simulink model "es2sim"  (R2023b)
settings: Solver=VariableStepAuto  StartTime=0.0  StopTime=200  RelTol=1e-3
values from neighbouring files (symbols this model uses):
  d = 0    [es2.m]
  ea0 = [0 0.3927 0]'    [es2.m]
  ea_dot_ref = [0.001745 0 0.04859]'    [es2.m]
  IJ = inv(J)    [es1.m]    (also in es2.m)
  J = diag([10000,9000,12000])    [es1.m]    (also in es2.m = [399 -2.81 -1.31)
  q0 = [0.6853,0.6953,0.1531,0.1531]'    [es1.m]    (also in es2.m = [0 0 1 0]')
  w0 = [0.53, 0.53,0.053]'    [es1.m]    (also in es2.m = [0.1 -0.9 0.12]')
libraries: vrlib x1
settings Model: Creator=luigi  LastModifiedBy=luigi

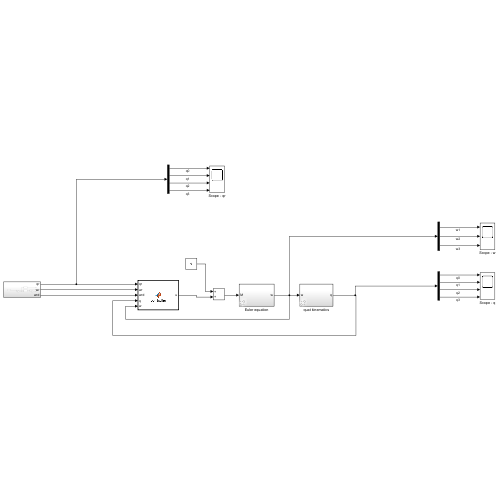
[thumbnail: Simulink's stored preview of the top-level diagram]
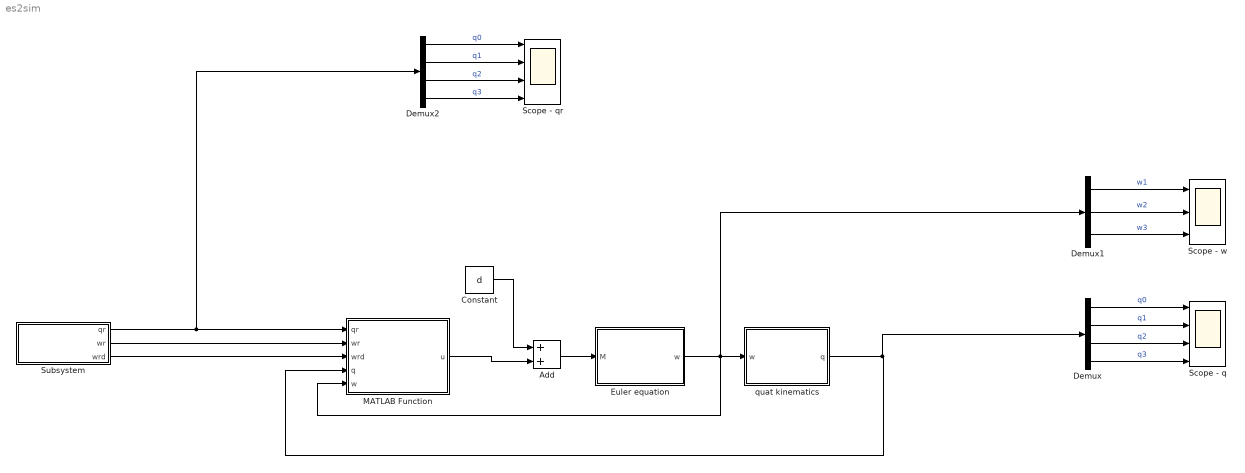
== system es2sim ==
  Add : Sum
  Constant : Constant  Value=d
  Demux : Demux
  Demux1 : Demux  Outputs=3
  Demux2 : Demux
  Euler equation : Subsystem  AncestorBlock=lib_rotations_2014/Euler equation
  MATLAB Function : MATLAB Function  TreatAsAtomicUnit=on
  Scope - q : Scope  NumInputPorts=4
  Scope - qr : Scope  NumInputPorts=4
  Scope - w : Scope  NumInputPorts=3
  Subsystem : Subsystem
  quat kinematics : Subsystem  AncestorBlock=lib_rotations_2014/quat kinematics
  wires:
  Add/1 -> Euler equation/1(M)
  Constant/1 -> Add/1
  MATLAB Function/1(u) -> Add/2
  Subsystem/2(wr) -> MATLAB Function/2(wr)
  Subsystem/3(wrd) -> MATLAB Function/3(wrd)
  Demux1/1 -> Scope - w/1  "w1"
  Demux1/2 -> Scope - w/2  "w2"
  Euler equation/1(w) -> Demux1/1, MATLAB Function/5(w), quat kinematics/1(w)
  Demux/2 -> Scope - q/2  "q1"
  Demux/4 -> Scope - q/4  "q3"
  Demux/1 -> Scope - q/1  "q0"
  Demux/3 -> Scope - q/3  "q2"
  Demux1/3 -> Scope - w/3  "w3"
  quat kinematics/1(q) -> Demux/1, MATLAB Function/4(q)
  Demux2/4 -> Scope - qr/4  "q3"
  Demux2/3 -> Scope - qr/3  "q2"
  Demux2/2 -> Scope - qr/2  "q1"
  Demux2/1 -> Scope - qr/1  "q0"
  Subsystem/1(qr) -> Demux2/1, MATLAB Function/1(qr)

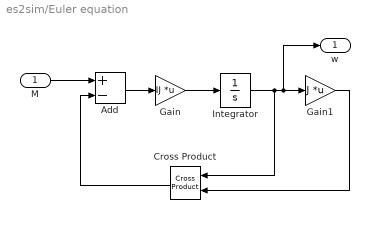
== system es2sim/Euler equation ==
  M : Inport
  Add : Sum  Inputs=+-
  Cross Product : vrlib/Utilities/Cross Product
  Gain : Gain  Gain=IJ  Multiplication=Matrix(K*u)
  Gain1 : Gain  Gain=J  Multiplication=Matrix(K*u)
  Integrator : Integrator  InitialCondition=w0
  w : Outport  PortDimensions=3  VectorParamsAs1DForOutWhenUnconnected=off
  wires:
  Cross Product/1 -> Add/2
  Add/1 -> Gain/1
  Gain1/1 -> Cross Product/2
  Gain/1 -> Integrator/1
  Integrator/1 -> Gain1/1, w/1, Cross Product/1
  M/1 -> Add/1

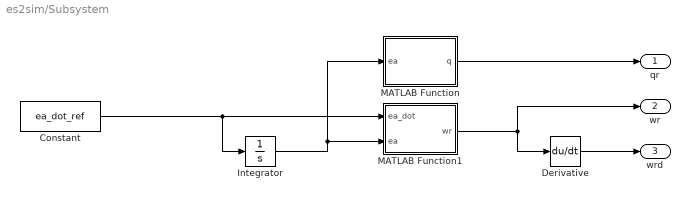
== system es2sim/Subsystem ==
  Constant : Constant  Value=ea_dot_ref
  Derivative : Derivative
  Integrator : Integrator  InitialCondition=ea0
  MATLAB Function : MATLAB Function  TreatAsAtomicUnit=on
  MATLAB Function1 : MATLAB Function  TreatAsAtomicUnit=on
  qr : Outport
  wr : Outport  Port=2
  wrd : Outport  Port=3
  wires:
  MATLAB Function/1(q) -> qr/1
  Constant/1 -> Integrator/1, MATLAB Function1/1(ea_dot)
  MATLAB Function1/1(wr) -> Derivative/1, wr/1
  Integrator/1 -> MATLAB Function/1(ea), MATLAB Function1/2(ea)
  Derivative/1 -> wrd/1

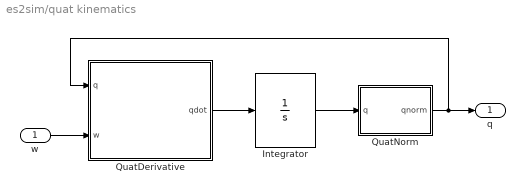
== system es2sim/quat kinematics ==
  w : Inport  PortDimensions=3
  Integrator : Integrator  InitialCondition=q0
  QuatDerivative : MATLAB Function  TreatAsAtomicUnit=on
  QuatNorm : MATLAB Function  TreatAsAtomicUnit=on
  q : Outport  PortDimensions=4  VectorParamsAs1DForOutWhenUnconnected=off
  wires:
  w/1 -> QuatDerivative/2(w)
  QuatDerivative/1(qdot) -> Integrator/1
  QuatNorm/1(qnorm) -> q/1, QuatDerivative/1(q)
  Integrator/1 -> QuatNorm/1(q)

== matlab function es2sim/quat kinematics/QuatDerivative ==
  data: q input; qdot output; w input
function qdot= QuatDerivative(q,w)
%#codegen
omegaq=[0; w];
Q=[q(1) -q(2) -q(3) -q(4);
    q(2) q(1) -q(4) q(3);
    q(3) q(4) q(1) -q(2);
    q(4) -q(3) q(2) q(1)];
qdot=Q*omegaq/2;

== matlab function es2sim/quat kinematics/QuatNorm ==
  data: q input; qnorm output
function qnorm = QuatNorm(q)
%#codegen
qnorm=zeros(4,1);
q2=sqrt(q'*q);
qnorm=q/q2;

== matlab function es2sim/MATLAB Function ==
  data: qr input; u output; wr input; wrd input; q input; w input
function u = controller(qr, wr, wrd, q, w)

w_tilde = wr - w;
q_star = [q(1);-q(2:4)]; q_tilde = quatprod(q_star,qr);

% Controller parameters
k1 = 1;
k2 = 1;
eta = 1;

J = [399 -2.81 -1.31;
    -2.81 377 2.54;
    -1.31 2.54 377];

s = w_tilde + k2*q_tilde(2:4); %sliding surface

% Linearization command
us = J*(wrd + (k2/2)*(q_tilde(1)*w_tilde + cross(q_tilde(2:4),(wr+w)))) + cross(w,J*w);

u = us + k1*J*tanh(eta*s);

end

function r = quatprod(q,p)

qq=[0 -q(4) q(3);
    q(4) 0 -q(2);
    -q(3) q(2) 0];

Q=[q(1) -q(2:4)'; 
    q(2:4) q(1)*eye(3)+qq];

r=Q*p;

end

== matlab function es2sim/Subsystem/MATLAB Function ==
  data: ea input; q output
function q = euler2quat(ea)
ph=ea(1);
th=ea(2);
ps=ea(3);


q1=[cos(ph/2);0;0;sin(ph/2)];
q2=[cos(th/2);sin(th/2);0;0];
q3=[cos(ps/2);0;0;sin(ps/2)];

q=quatprod(q1,quatprod(q2,q3));
end

function r=quatprod(q,p)

qq=[0 -q(4) q(3);
    q(4) 0 -q(2);
    -q(3) q(2) 0];

Q=[q(1) -q(2:4)'; 
    q(2:4) q(1)*eye(3)+qq];

r=Q*p;

end

== matlab function es2sim/Subsystem/MATLAB Function1 ==
  data: ea_dot input; ea input; wr output
function wr = kin_eq(ea_dot, ea)

ph = ea(1);
th = ea(2); 
ps = ea(3);

T = [sin(th)*sin(ps) cos(ps) 0;
    sin(th)*cos(ps) -sin(ps) 0;
    cos(th) 0 1];    
   
wr = T*ea_dot;
end
